simulink model "elec_auto_ev"  (R2017b)
settings: Solver=FixedStepAuto  StartTime=0.0  StopTime=200  RelTol=1e-3  AbsTol=1e-3
PreLoadFcn:
  | % Simulation parameters
  | dt = 0.01;
  | 
  | % Battery cell parameters
  | ssc_lithium_cell_1RC_ini
  | 
  | % Motor parameters
  | max_torque = 220;
  | max_power = 50e3;
  | 
  | % Vehicle parameters
  | vehicle_mass = 1000;
  | wheel_radius = 0.25;
  | area = 5;
  | drag_coefficient = 0.25;
  | air_density = 1.225;
  | gravity = 9.81;
  | rolling_res_ratio = 0.015;
  | 
  | % Differential drive parameters
  | gear_ratio = 6;
  | 
  | % Simplified braking system parameters
  | force_max_pedal = 500;
  | braking_torque_to_pedal_force_ratio = -4;
  | 
  | % Vehicle controller parameters
  | hill_hold_max_speed = 0.5;
  | 
  | % Water properties for cooling circuit
  | load WaterProperties
undefined symbols (not defined in the file): C1_LUT, Capacity_LUT, cell_Cp_heat, cell_mass, DiscIntNeverNeededParam, Em_LUT, Qe_init, R0_LUT, R1_LUT, sigbuilder_block, SOC_LUT, T_init, Temperature_LUT
libraries: fl_lib x93, nesl_utility x12, LiBatteryElements_lib x4, elec_lib x2, simulink x2, simulink_extras x1
(part 2 of 2)

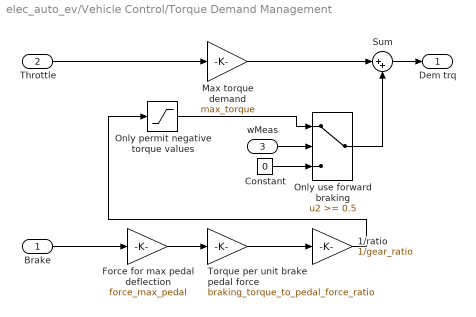
== system elec_auto_ev/Vehicle Control/Torque Demand Management ==
  Brake : Inport
  Throttle : Inport  Port=2
  wMeas : Inport  Port=3
  1/ratio : Gain  Gain=1/gear_ratio
  Constant : Constant  Value=0  SampleTime=dt
  Force for max pedal deflection : Gain  Gain=force_max_pedal
  Max torque demand : Gain  Gain=max_torque
  Only permit negative torque values : Saturate  UpperLimit=-10  LowerLimit=-max_torque
  Only use forward braking : Switch  Threshold=0.5  InputSameDT=on
  Sum : Sum  Inputs=|++
  Torque per unit brake pedal force : Gain  Gain=braking_torque_to_pedal_force_ratio
  Dem trq : Outport
  wires:
  Max torque demand/1 -> Sum/1
  Brake/1 -> Force for max pedal deflection/1
  Sum/1 -> Dem trq/1
  Throttle/1 -> Max torque demand/1
  Torque per unit brake pedal force/1 -> 1/ratio/1
  1/ratio/1 -> Only permit negative torque values/1
  Force for max pedal deflection/1 -> Torque per unit brake pedal force/1
  wMeas/1 -> Only use forward braking/2
  Only use forward braking/1 -> Sum/2
  Constant/1 -> Only use forward braking/3
  Only permit negative torque values/1 -> Only use forward braking/1

== system elec_auto_ev/Battery/Electric and Thermal Model/Thermal Model ==
  Battery Thermal Mass : fl_lib/Thermal/Thermal Elements/Thermal Mass  mass=cell_mass*Nseries*Nparallel kg  sp_heat=cell_Cp_heat J/kg/K  T_specify=on  T_priority=High  T=T_init K  T_nominal_specify=off  T_nominal_unit=K  T_nominal_value=1  Q_specify=off  Q_priority=High  Q=0 J/s  Q_nominal_specify=off  Q_nominal_unit=J/s  Q_nominal_value=1
      settings: SourceProductName=Foundation Library
  Heat Flow Source : fl_lib/Thermal/Thermal Sources/Controlled Heat Flow Rate Source
      settings: SourceProductName=Foundation Library
  Ideal Temperature Sensor : fl_lib/Thermal/Thermal Sensors/Temperature Sensor
      settings: SourceProductName=Foundation Library
  ThRef1 : fl_lib/Thermal/Thermal Elements/Thermal Reference
      settings: SourceProductName=Foundation Library
  ThRef2 : fl_lib/Thermal/Thermal Elements/Thermal Reference
      settings: SourceProductName=Foundation Library
  PlossTotal : PMIOPort  Tag=PMCPort  Port=1  Side=Left
  T : PMIOPort  Tag=PMCPort  Port=2  Side=Right
  H : PMIOPort  Tag=PMCPort  Port=3  Side=Left
  connections:
  ThRef2/LConn1 -- Ideal Temperature Sensor/RConn1
  Ideal Temperature Sensor/RConn2 -- T/RConn1
  ThRef1/LConn1 -- Heat Flow Source/RConn2
  Ideal Temperature Sensor/LConn1 -- H/RConn1 -- Battery Thermal Mass/LConn1 -- Heat Flow Source/LConn1
  Heat Flow Source/RConn1 -- PlossTotal/RConn1

== system elec_auto_ev/Cooling System/Heat Exch. Characteristic/Characteristic ==
  PS Product : fl_lib/Physical Signals/Functions/PS Product
      settings: SourceProductName=Foundation Library
  PS Subtract : fl_lib/Physical Signals/Functions/PS Subtract
      settings: SourceProductName=Foundation Library
  Specific dissipation (J/s/K) per unit mass flow rate : fl_lib/Physical Signals/Functions/PS Gain  gain=100
      settings: SourceProductName=Foundation Library
  M : PMIOPort  Port=1  Side=Right
  T in : PMIOPort  Port=2  Side=Right
  T Env : PMIOPort  Port=3  Side=Right
  Q : PMIOPort  Port=4  Side=Left
  connections:
  T Env/RConn1 -- PS Subtract/LConn1
  PS Product/RConn1 -- Q/RConn1
  PS Subtract/RConn1 -- PS Product/LConn1
  T in/RConn1 -- PS Subtract/LConn2
  M/RConn1 -- Specific dissipation (J/s/K) per unit mass flow rate/LConn1
  PS Product/LConn2 -- Specific dissipation (J/s/K) per unit mass flow rate/RConn1

== system elec_auto_ev/PMSM Drive/Heat Exch. Characteristic/Characteristic ==
  PS Product : fl_lib/Physical Signals/Functions/PS Product
      settings: SourceProductName=Foundation Library
  PS Subtract : fl_lib/Physical Signals/Functions/PS Subtract
      settings: SourceProductName=Foundation Library
  Specific dissipation (J/s/K) : fl_lib/Physical Signals/Lookup Tables/PS Lookup Table (1D)  x="[0 0.2 0.4  0.7  1 1.2  1.4  2.5 ]"  f=100 * [0 0.5 0.75 0.92 1 1.02 1.03 1.04]  interp_method=1  extrap_method=1
      settings: SourceProductName=Foundation Library
  Specific dissipation (J/s/K) per unit mass flow rate : fl_lib/Physical Signals/Functions/PS Gain  gain=100
      settings: SourceProductName=Foundation Library
  Mass Flow : PMIOPort  Port=1  Side=Left
  Temp Inlet : PMIOPort  Port=2  Side=Left
  Temp Motor : PMIOPort  Port=3  Side=Left
  Q : PMIOPort  Port=4  Side=Right
  connections:
  PS Subtract/RConn1 -- PS Product/LConn1
  Specific dissipation (J/s/K)/RConn1 -- PS Product/LConn2
  Temp Motor/RConn1 -- PS Subtract/LConn1
  PS Subtract/LConn2 -- Temp Inlet/RConn1
  PS Product/RConn1 -- Q/RConn1
  Mass Flow/RConn1 -- Specific dissipation (J/s/K) per unit mass flow rate/LConn1
  Specific dissipation (J/s/K) per unit mass flow rate/RConn1 -- Specific dissipation (J/s/K)/LConn1

== system elec_auto_ev/Vehicle Dynamics/Brake Torque/Smooth Sign ==
  1 : fl_lib/Physical Signals/Sources/PS Constant  constant=1
      settings: SourceProductName=Foundation Library
  2 : fl_lib/Physical Signals/Functions/PS Gain  gain=2
      settings: SourceProductName=Foundation Library
  exp(2x) : fl_lib/Physical Signals/Functions/PS Math Function  fcn_choice=3
      settings: SourceProductName=Foundation Library
  exp(2x)+1 : fl_lib/Physical Signals/Functions/PS Add
      settings: SourceProductName=Foundation Library
  exp(2x)-1 : fl_lib/Physical Signals/Functions/PS Subtract
      settings: SourceProductName=Foundation Library
  tanh(x) : fl_lib/Physical Signals/Functions/PS Divide
      settings: SourceProductName=Foundation Library
  x : PMIOPort  Port=1  Side=Left
  y : PMIOPort  Port=2  Side=Right
  connections:
  y/RConn1 -- tanh(x)/RConn1
  x/RConn1 -- 2/LConn1
  exp(2x)-1/RConn1 -- tanh(x)/LConn1
  exp(2x)+1/RConn1 -- tanh(x)/LConn2
  exp(2x)+1/LConn2 -- exp(2x)-1/LConn1 -- exp(2x)/RConn1
  2/RConn1 -- exp(2x)/LConn1
  exp(2x)-1/LConn2 -- exp(2x)+1/LConn1 -- 1/RConn1

== system elec_auto_ev/Vehicle Dynamics/Drag and Gravity/Smooth Step ==
  1 : fl_lib/Physical Signals/Sources/PS Constant  constant=1
      settings: SourceProductName=Foundation Library
  2 : fl_lib/Physical Signals/Functions/PS Gain  gain=2
      settings: SourceProductName=Foundation Library
  exp(2x) : fl_lib/Physical Signals/Functions/PS Math Function  fcn_choice=3
      settings: SourceProductName=Foundation Library
  exp(2x)+1 : fl_lib/Physical Signals/Functions/PS Add
      settings: SourceProductName=Foundation Library
  exp(2x)-1 : fl_lib/Physical Signals/Functions/PS Subtract
      settings: SourceProductName=Foundation Library
  tanh(x) : fl_lib/Physical Signals/Functions/PS Divide
      settings: SourceProductName=Foundation Library
  x : PMIOPort  Port=1  Side=Left
  y : PMIOPort  Port=2  Side=Right
  connections:
  y/RConn1 -- tanh(x)/RConn1
  x/RConn1 -- 2/LConn1
  exp(2x)-1/RConn1 -- tanh(x)/LConn1
  exp(2x)+1/RConn1 -- tanh(x)/LConn2
  exp(2x)+1/LConn2 -- exp(2x)-1/LConn1 -- exp(2x)/RConn1
  2/RConn1 -- exp(2x)/LConn1
  exp(2x)-1/LConn2 -- exp(2x)+1/LConn1 -- 1/RConn1

== system elec_auto_ev/Vehicle Control/Cruise Control/Capture speed ==
  In1 : Inport
  Trigger : TriggerPort  VariantControl=Variant
  Out1 : Outport
  wires:
  In1/1 -> Out1/1

== system elec_auto_ev/Vehicle Control/Cruise Control/Speed Controller ==
  wRef : Inport
  wMeas : Inport  Port=2
  Add : Sum  Inputs=|+-
  Add1 : Sum
  Discrete-Time Integrator : DiscreteIntegrator  gainval=Ki  SampleTime=ts  LimitOutput=on  UpperSaturationLimit=trqMax  LowerSaturationLimit=-trqMax  ICPrevOutput=DiscIntNeverNeededParam  ICPrevScaledInput=DiscIntNeverNeededParam
  Kp : Gain  Gain=Kp
  trqRef : Outport
  wires:
  wRef/1 -> Add/1
  Kp/1 -> Add1/1
  Discrete-Time Integrator/1 -> Add1/2
  wMeas/1 -> Add/2
  Add1/1 -> trqRef/1
  Add/1 -> Kp/1, Discrete-Time Integrator/1
